simulink model "Hybrid2_article_SVC_stage1"  (R2025a)
settings: Solver=FixedStepAuto  StartTime=0.0  StopTime=0.2  FixedStep=Ts  RelTol=1e-3
undefined symbols (not defined in the file or in its folder): closedLoop, controller, D1, D11, Delta, DiscIntNeverNeededParam, find_system, grid, level, protection, sensor, solarPanel, solarPlant, Ts
libraries: powerlib_extras x38, nesl_utility x29, spsSampleandHoldLib x24, spsThyristorLib x24, spsSeriesRLCBranchLib x23, simulink x22, fl_lib x18, ee_lib x12, spsEdgeDetectorLib x12, spsParallelRLCBranchLib x10, spsThreePhaseVIMeasurementLib x9, simulink_extras x8
(part 7 of 8)

== system Hybrid2_article_SVC_stage1/SVC Controller1/Firing Unit/Firing Unit BC/TCR Pulse Generatorr ==
  Ns/c : Inport
  Alpha : Inport  Port=2  PortDimensions=1
  Sync +/- : Inport  Port=3  PortDimensions=1
  SqWave : Inport  Port=4  PortDimensions=1
  Alpha 90<A<181 : Constant  Value=90
  Alpha 90<A<182 : Constant  Value=360
  Alpha 90<A<183 : Constant  Value=2
  Alpha 90<A<184 : Constant  Value=2
  Alpha 90<A<185 : Constant  Value=87
  Data Type Conversion : DataTypeConversion  OutDataTypeStr=double  SaturateOnIntegerOverflow=off  RndMeth=Floor
  Discrete-Time Integrator : DiscreteIntegrator  ExternalReset=rising  SampleTime=Ts  LimitOutput=on  UpperSaturationLimit=100000  LowerSaturationLimit=0  ICPrevOutput=DiscIntNeverNeededParam  ICPrevScaledInput=DiscIntNeverNeededParam
  Gain2 : Gain  Gain=1/Ts  OutDataTypeStr=double  SaturateOnIntegerOverflow=on  ParamDataTypeStr=Inherit: Same as input
  Logical Operator1 : Logic  Inputs=3
  Logical Operator2 : Logic  Operator=NOT  Inputs=3
  Product : Product  Inputs=*/  InputSameDT=on  SaturateOnIntegerOverflow=on  OutDataTypeStr=Inherit: Same as first input
  Product1 : Product  Inputs=**  InputSameDT=on  SaturateOnIntegerOverflow=on  OutDataTypeStr=Inherit: Same as first input
  Product2 : Product  Inputs=*/  InputSameDT=on  SaturateOnIntegerOverflow=on  OutDataTypeStr=Inherit: Same as first input
  Relational Operator1 : RelationalOperator  Operator=<=
  Relational Operator2 : RelationalOperator
  Relational Operator3 : RelationalOperator  Operator=<=
  Rounding Function1 : Rounding  Operator=round
  Rounding Function3 : Rounding  Operator=round
  Sample and Hold : spsSampleandHoldLib/Sample and Hold  ic=180  Ts=Ts
      settings: AttributesFormatString=IC = %<ic>
  Sum1 : Sum  Inputs=+-  InputSameDT=on  SaturateOnIntegerOverflow=on  OutDataTypeStr=Inherit: Same as first input
  Sum2 : Sum  Inputs=+--  InputSameDT=on  SaturateOnIntegerOverflow=on  OutDataTypeStr=Inherit: Same as first input
  Switch : Switch  Criteria=u2 > Threshold
  TCR +/- : Outport  VectorParamsAs1DForOutWhenUnconnected=off
  wires:
  Alpha 90<A<181/1 -> Sum1/2
  Ns/c/1 -> Product1/1, Product2/1
  Product1/1 -> Rounding Function1/1
  Alpha 90<A<182/1 -> Product/2
  Product/1 -> Product1/2
  Product2/1 -> Rounding Function3/1
  Alpha 90<A<183/1 -> Product2/2
  Sum1/1 -> Product/1, Relational Operator1/1
  Alpha 90<A<185/1 -> Relational Operator1/2
  Alpha/1 -> Sample and Hold/1
  Rounding Function1/1 -> Sum2/3, Switch/1
  Rounding Function3/1 -> Sum2/1, Switch/3
  Alpha 90<A<184/1 -> Sum2/2
  Relational Operator1/1 -> Switch/2
  Relational Operator3/1 -> Logical Operator1/3
  Discrete-Time Integrator/1 -> Relational Operator2/1, Relational Operator3/1
  Relational Operator2/1 -> Logical Operator1/2
  Logical Operator1/1 -> TCR +/-/1
  Switch/1 -> Relational Operator2/2
  Sum2/1 -> Relational Operator3/2
  Logical Operator2/1 -> Discrete-Time Integrator/2
  SqWave/1 -> Data Type Conversion/1, Logical Operator2/1, Logical Operator1/1
  Sync +/-/1 -> Sample and Hold/2
  Sample and Hold/1 -> Sum1/1
  Data Type Conversion/1 -> Gain2/1
  Gain2/1 -> Discrete-Time Integrator/1

== system Hybrid2_article_SVC_stage1/SVC Controller1/Firing Unit/Firing Unit BC/TCR Pulse Generatorr1 ==
  Ns/c : Inport
  Alpha : Inport  Port=2  PortDimensions=1
  Sync +/- : Inport  Port=3  PortDimensions=1
  SqWave : Inport  Port=4  PortDimensions=1
  Alpha 90<A<181 : Constant  Value=90
  Alpha 90<A<182 : Constant  Value=360
  Alpha 90<A<183 : Constant  Value=2
  Alpha 90<A<184 : Constant  Value=2
  Alpha 90<A<185 : Constant  Value=87
  Data Type Conversion : DataTypeConversion  OutDataTypeStr=double  SaturateOnIntegerOverflow=off  RndMeth=Floor
  Discrete-Time Integrator : DiscreteIntegrator  ExternalReset=rising  SampleTime=Ts  OutDataTypeStr=double  LimitOutput=on  UpperSaturationLimit=100000  LowerSaturationLimit=0  ICPrevOutput=DiscIntNeverNeededParam  ICPrevScaledInput=DiscIntNeverNeededParam
  Gain2 : Gain  Gain=1/Ts  OutDataTypeStr=double  ParamDataTypeStr=Inherit: Same as input
  Logical Operator1 : Logic  Inputs=3
  Logical Operator2 : Logic  Operator=NOT  Inputs=3
  Product : Product  Inputs=*/  InputSameDT=on  SaturateOnIntegerOverflow=on  OutDataTypeStr=Inherit: Same as first input
  Product1 : Product  Inputs=**  InputSameDT=on  SaturateOnIntegerOverflow=on  OutDataTypeStr=Inherit: Same as first input
  Product2 : Product  Inputs=*/  InputSameDT=on  SaturateOnIntegerOverflow=on  OutDataTypeStr=Inherit: Same as first input
  Relational Operator1 : RelationalOperator  Operator=<=
  Relational Operator2 : RelationalOperator
  Relational Operator3 : RelationalOperator  Operator=<=
  Rounding Function1 : Rounding  Operator=round
  Rounding Function3 : Rounding  Operator=round
  Sample and Hold : spsSampleandHoldLib/Sample and Hold  ic=180  Ts=Ts
      settings: AttributesFormatString=IC = %<ic>
  Sum1 : Sum  Inputs=+-  InputSameDT=on  SaturateOnIntegerOverflow=on  OutDataTypeStr=Inherit: Same as first input
  Sum2 : Sum  Inputs=+--  OutDataTypeStr=Inherit: Inherit via back propagation  InputSameDT=on  SaturateOnIntegerOverflow=on
  Switch : Switch  Criteria=u2 > Threshold  OutDataTypeStr=Inherit: Inherit via back propagation
  TCR +/- : Outport  VectorParamsAs1DForOutWhenUnconnected=off
  wires:
  Alpha 90<A<181/1 -> Sum1/2
  Ns/c/1 -> Product1/1, Product2/1
  Product1/1 -> Rounding Function1/1
  Alpha 90<A<182/1 -> Product/2
  Product/1 -> Product1/2
  Product2/1 -> Rounding Function3/1
  Alpha 90<A<183/1 -> Product2/2
  Sum1/1 -> Product/1, Relational Operator1/1
  Alpha 90<A<185/1 -> Relational Operator1/2
  Alpha/1 -> Sample and Hold/1
  Rounding Function1/1 -> Sum2/3, Switch/1
  Rounding Function3/1 -> Sum2/1, Switch/3
  Alpha 90<A<184/1 -> Sum2/2
  Relational Operator1/1 -> Switch/2
  Relational Operator3/1 -> Logical Operator1/3
  Discrete-Time Integrator/1 -> Relational Operator2/1, Relational Operator3/1
  Relational Operator2/1 -> Logical Operator1/2
  Logical Operator1/1 -> TCR +/-/1
  Gain2/1 -> Discrete-Time Integrator/1
  Switch/1 -> Relational Operator2/2
  Sum2/1 -> Relational Operator3/2
  Logical Operator2/1 -> Discrete-Time Integrator/2
  SqWave/1 -> Data Type Conversion/1, Logical Operator1/1, Logical Operator2/1
  Sync +/-/1 -> Sample and Hold/2
  Sample and Hold/1 -> Sum1/1
  Data Type Conversion/1 -> Gain2/1

== system Hybrid2_article_SVC_stage1/SVC Controller1/Firing Unit/Firing Unit BC/TCS Pulse Generator ==
  note: Note: Sync+ , Sync - and SqWave signals are inverted for TSC firing (i.e. positive thyristor is fired on negative peak voltage)
  SqWave : Inport  PortDimensions=1
  Sync + : Inport  Port=2  PortDimensions=1
  Sync - : Inport  Port=3  PortDimensions=1
  TSC_On : Inport  Port=4  PortDimensions=1
  Alpha1 : Constant  Value=FiringMode-1  OutDataTypeStr=Inherit: Inherit via back propagation
  Delay : Delay  DelayLength=fix(1/FreqInit/Ts)
  Logical Operator1 : Logic  Operator=NOT
  Logical Operator10 : Logic  Operator=OR
  Logical Operator11 : Logic  Inputs=3
  Logical Operator12 : Logic
  Logical Operator13 : Logic
  Logical Operator14 : Logic  Operator=OR
  Logical Operator15 : Logic  Inputs=3
  Sample and Hold : spsSampleandHoldLib/Sample and Hold  ic=0  Ts=Ts
      settings: AttributesFormatString=IC = %<ic>
  Sample and Hold1 : spsSampleandHoldLib/Sample and Hold  ic=0  Ts=Ts
      settings: AttributesFormatString=IC = %<ic>
  TSC + : Outport  VectorParamsAs1DForOutWhenUnconnected=off
  TSC - : Outport  Port=2  VectorParamsAs1DForOutWhenUnconnected=off
  wires:
  Delay/1 -> Logical Operator14/2, Logical Operator10/2
  Logical Operator15/1 -> TSC -/1
  Logical Operator11/1 -> TSC +/1
  Logical Operator14/1 -> Logical Operator15/2
  Logical Operator10/1 -> Logical Operator11/2
  Logical Operator1/1 -> Logical Operator10/1
  SqWave/1 -> Logical Operator14/1, Logical Operator1/1
  Logical Operator12/1 -> Delay/1
  Alpha1/1 -> Logical Operator12/2
  Logical Operator13/1 -> Logical Operator12/1
  TSC_On/1 -> Sample and Hold1/1, Sample and Hold/1, Logical Operator15/3, Logical Operator11/3
  Sync -/1 -> Sample and Hold/2
  Sync +/1 -> Sample and Hold1/2
  Sample and Hold/1 -> Logical Operator13/1, Logical Operator11/1
  Sample and Hold1/1 -> Logical Operator13/2, Logical Operator15/1

== system Hybrid2_article_SVC_stage1/SVC Controller1/Firing Unit/Firing Unit BC/TCS Pulse Generator1 ==
  note: Note: Sync+ , Sync - and SqWave signals are inverted for TSC firing (i.e. positive thyristor is fired on negative peak voltage)
  SqWave : Inport  PortDimensions=1
  Sync + : Inport  Port=2  PortDimensions=1
  Sync - : Inport  Port=3  PortDimensions=1
  TSC_On : Inport  Port=4  PortDimensions=1
  Alpha1 : Constant  Value=FiringMode-1
  Data Type Conversion : DataTypeConversion  OutDataTypeStr=boolean  SaturateOnIntegerOverflow=off  RndMeth=Floor
  Delay : Delay  DelayLength=fix(1/FreqInit/Ts)
  Logical Operator1 : Logic  Operator=NOT
  Logical Operator10 : Logic  Operator=OR
  Logical Operator11 : Logic  Inputs=3
  Logical Operator12 : Logic
  Logical Operator13 : Logic
  Logical Operator14 : Logic  Operator=OR
  Logical Operator15 : Logic  Inputs=3
  Sample and Hold : spsSampleandHoldLib/Sample and Hold  ic=0  Ts=Ts
      settings: AttributesFormatString=IC = %<ic>
  Sample and Hold1 : spsSampleandHoldLib/Sample and Hold  ic=0  Ts=Ts
      settings: AttributesFormatString=IC = %<ic>
  TSC + : Outport  VectorParamsAs1DForOutWhenUnconnected=off
  TSC - : Outport  Port=2  VectorParamsAs1DForOutWhenUnconnected=off
  wires:
  Delay/1 -> Logical Operator14/2, Logical Operator10/2
  Logical Operator15/1 -> TSC -/1
  Logical Operator11/1 -> TSC +/1
  Logical Operator14/1 -> Logical Operator15/2
  Logical Operator10/1 -> Logical Operator11/2
  Logical Operator1/1 -> Logical Operator10/1
  SqWave/1 -> Logical Operator14/1, Logical Operator1/1
  Logical Operator12/1 -> Delay/1
  Logical Operator13/1 -> Logical Operator12/1
  TSC_On/1 -> Sample and Hold1/1, Sample and Hold/1, Logical Operator15/3, Logical Operator11/3
  Sync -/1 -> Sample and Hold/2
  Sync +/1 -> Sample and Hold1/2
  Sample and Hold/1 -> Logical Operator13/1, Logical Operator11/1
  Sample and Hold1/1 -> Logical Operator13/2, Logical Operator15/1
  Alpha1/1 -> Data Type Conversion/1
  Data Type Conversion/1 -> Logical Operator12/2

== system Hybrid2_article_SVC_stage1/SVC Controller1/Firing Unit/Firing Unit BC/TCS Pulse Generator2 ==
  note: Note: Sync+ , Sync - and SqWave signals are inverted for TSC firing (i.e. positive thyristor is fired on negative peak voltage)
  SqWave : Inport  PortDimensions=1
  Sync + : Inport  Port=2  PortDimensions=1
  Sync - : Inport  Port=3  PortDimensions=1
  TSC_On : Inport  Port=4  PortDimensions=1
  Alpha1 : Constant  Value=FiringMode-1
  Data Type Conversion : DataTypeConversion  OutDataTypeStr=boolean  SaturateOnIntegerOverflow=off  RndMeth=Floor
  Delay : Delay  DelayLength=fix(1/FreqInit/Ts)
  Logical Operator1 : Logic  Operator=NOT
  Logical Operator10 : Logic  Operator=OR
  Logical Operator11 : Logic  Inputs=3
  Logical Operator12 : Logic
  Logical Operator13 : Logic
  Logical Operator14 : Logic  Operator=OR
  Logical Operator15 : Logic  Inputs=3
  Sample and Hold : spsSampleandHoldLib/Sample and Hold  ic=0  Ts=Ts
      settings: AttributesFormatString=IC = %<ic>
  Sample and Hold1 : spsSampleandHoldLib/Sample and Hold  ic=0  Ts=Ts
      settings: AttributesFormatString=IC = %<ic>
  TSC + : Outport  VectorParamsAs1DForOutWhenUnconnected=off
  TSC - : Outport  Port=2  VectorParamsAs1DForOutWhenUnconnected=off
  wires:
  Delay/1 -> Logical Operator14/2, Logical Operator10/2
  Logical Operator15/1 -> TSC -/1
  Logical Operator11/1 -> TSC +/1
  Logical Operator14/1 -> Logical Operator15/2
  Logical Operator10/1 -> Logical Operator11/2
  Logical Operator1/1 -> Logical Operator10/1
  SqWave/1 -> Logical Operator14/1, Logical Operator1/1
  Logical Operator12/1 -> Delay/1
  Alpha1/1 -> Data Type Conversion/1
  Logical Operator13/1 -> Logical Operator12/1
  TSC_On/1 -> Sample and Hold1/1, Sample and Hold/1, Logical Operator15/3, Logical Operator11/3
  Sync -/1 -> Sample and Hold/2
  Sync +/1 -> Sample and Hold1/2
  Sample and Hold/1 -> Logical Operator13/1, Logical Operator11/1
  Sample and Hold1/1 -> Logical Operator13/2, Logical Operator15/1
  Data Type Conversion/1 -> Logical Operator12/2

== system Hybrid2_article_SVC_stage1/SVC Controller1/Firing Unit/Firing Unit CA/BL2 ==
  Freq : Inport  PortDimensions=1
  Constant1 : Constant  Value=0
  Constant2 : Constant  Value=1e-5
  Constant3 : Constant
  Gain : Gain  Gain=Ts  SaturateOnIntegerOverflow=on  OutDataTypeStr=Inherit: Same as input  ParamDataTypeStr=Inherit: Same as input
  Product : Product  Inputs=/*  InputSameDT=on  SaturateOnIntegerOverflow=on  OutDataTypeStr=Inherit: Same as first input
  Relational Operator1 : RelationalOperator  Operator=~=
  Switch : Switch  Threshold=0.5
  Ns/c : Outport  VectorParamsAs1DForOutWhenUnconnected=off
  wires:
  Product/1 -> Ns/c/1
  Freq/1 -> Gain/1
  Constant1/1 -> Relational Operator1/2
  Gain/1 -> Relational Operator1/1, Switch/1
  Constant2/1 -> Switch/3
  Relational Operator1/1 -> Switch/2
  Switch/1 -> Product/1
  Constant3/1 -> Product/2

== system Hybrid2_article_SVC_stage1/SVC Controller1/Firing Unit/Firing Unit CA/BL3 ==
  Freq : Inport  PortDimensions=1
  sin(wt) : Inport  Port=2  PortDimensions=1
  Bistable : spsBistableLib/Bistable  Qpriority=Set  ic=0  Ts=Ts
  Data Type Conversion : DataTypeConversion  SaturateOnIntegerOverflow=off  RndMeth=Floor
  Edge Detector : spsEdgeDetectorLib/Edge Detector  model=Rising  ic=0  Ts=Ts
  Edge Detector1 : spsEdgeDetectorLib/Edge Detector  model=Falling  ic=0  Ts=Ts
  Edge Detector2 : spsEdgeDetectorLib/Edge Detector  model=Rising  ic=0  Ts=Ts
  Edge Detector3 : spsEdgeDetectorLib/Edge Detector  model=Rising  ic=0  Ts=Ts
  Product2 : Product  InputSameDT=on  SaturateOnIntegerOverflow=on  OutDataTypeStr=Inherit: Same as first input
  Relational Operator : RelationalOperator  Operator=>
  Relational Operator2 : RelationalOperator  Operator=<
  Sum5 : Sum  Inputs=+-  InputSameDT=on  SaturateOnIntegerOverflow=on  OutDataTypeStr=Inherit: Same as first input
  Sum6 : Sum  InputSameDT=on  SaturateOnIntegerOverflow=on  OutDataTypeStr=Inherit: Same as first input
  Terminator : Terminator
  Trigonometric Function7 : Trigonometry
  alpha2 : Constant  Value=0
  alpha9 : Constant  Value=pi*Ts
  SqWave : Outport  VectorParamsAs1DForOutWhenUnconnected=off
  Sync + : Outport  Port=2  VectorParamsAs1DForOutWhenUnconnected=off
  Sync - : Outport  Port=3  VectorParamsAs1DForOutWhenUnconnected=off
  wires:
  Data Type Conversion/1 -> Edge Detector/1, Edge Detector1/1, SqWave/1
  Bistable/2 -> Terminator/1
  Edge Detector3/1 -> Bistable/2
  Edge Detector2/1 -> Bistable/1
  Edge Detector1/1 -> Sync -/1
  Edge Detector/1 -> Sync +/1
  Bistable/1 -> Data Type Conversion/1
  alpha9/1 -> Product2/1
  Product2/1 -> Trigonometric Function7/1
  Relational Operator2/1 -> Edge Detector3/1
  Relational Operator/1 -> Edge Detector2/1
  Sum6/1 -> Relational Operator2/2
  Sum5/1 -> Relational Operator/2
  alpha2/1 -> Sum6/1, Sum5/1
  Trigonometric Function7/1 -> Sum6/2, Sum5/2
  Freq/1 -> Product2/2
  sin(wt)/1 -> Relational Operator/1, Relational Operator2/1

== system Hybrid2_article_SVC_stage1/SVC Controller1/Firing Unit/Firing Unit CA/PLL sync on positive peak  ==
  note: Note: -sin( a ) * sin( b ) = 1/2 * cos( a+b ) - 1/2 * cos(a-b)
  note: Discrete 1-phase PLL
  note: Note: PLL synchronized on positive peak of input
  note: Pierre Giroux, Gilbert Sybille
      | Power System Laboratory, IREQ
      | Hydro-Quebec
  V(pu) : Inport
  Constant4 : Constant  Value=2*pi
  Discrete PI Controller : Subsystem  DialogController=POWERSYS.PowerSysDialog  mask(Discrete PI Controller){Kp=Kp, Ki=Ki, Par_Limits=[1.25  0.75]*2*pi*Finit, Init=2*pi*Finit, Ts=Ts}
      mask prompts: Kp "Proportional gain (Kp):"; Ki "Integral gain (Ki):"; Par_Limits "Output limits: [ Upper   Lower ]"; Init "Output initial value:"; Ts "Sample time:"
      mask help: This block implements a discrete PI controller.
      mask init:
      | UpperLimit=Par_Limits(1);
      | LowerLimit=Par_Limits(2);
      | power_initmask();
      mask Help: This block is part of a subset of blocks in the Extras library that does not have documentation associated with it, other than the block mask description.
      mask Display: disp('PI');
  Discrete-Time Integrator : DiscreteIntegrator  InitialCondition=(Phase_Init-90)*pi/180  SampleTime=Ts  ICPrevOutput=DiscIntNeverNeededParam  ICPrevScaledInput=DiscIntNeverNeededParam
  Gain10 : Gain  Gain=1/2/pi  SaturateOnIntegerOverflow=on  OutDataTypeStr=Inherit: Same as input  ParamDataTypeStr=Inherit: Same as input
  Gain12 : Gain  Gain=-1  SaturateOnIntegerOverflow=on  OutDataTypeStr=Inherit: Same as input  ParamDataTypeStr=Inherit: Same as input
  Math Function : Math  Operator=mod  SignedPower=on
  Mean (Variable Frequency)1 : spsMeanVariableFrequencyLib/Mean (Variable Frequency)  Finit=Finit  Fmin=45  Vinit=0  Ts=Ts
  Product1 : Product  InputSameDT=on  SaturateOnIntegerOverflow=on  OutDataTypeStr=Inherit: Same as first input
  Rate Limiter : RateLimiter  RisingSlewLimit=10  FallingSlewLimit=-10  SampleTimeMode=inherited  InitialCondition=Finit
  Second-Order Filter : spsSecondOrderFilterLib/Second-Order Filter  FilterType=Lowpass  Fo=25  Zeta=0.707  Ts=Ts  Initialize=on  Vac_Init="[0 0  Finit]"  Vdc_Init=Finit  PlotResponse=off  FreqRange=[1 500 1]
  Trigonometric Function6 : Trigonometry
  Unit Delay1 : UnitDelay  InitialCondition=Finit  SampleTime=Ts  HasFrameUpgradeWarning=on
      settings: AttributesFormatString=IC = %<InitialCondition>
  Freq : Outport  VectorParamsAs1DForOutWhenUnconnected=off
  wt : Outport  Port=2  VectorParamsAs1DForOutWhenUnconnected=off
  wires:
  Gain12/1 -> Product1/1
  V(pu)/1 -> Gain12/1
  Constant4/1 -> Math Function/2
  Discrete-Time Integrator/1 -> Math Function/1
  Product1/1 -> Mean (Variable Frequency)1/2
  Discrete PI Controller/1(Out) -> Discrete-Time Integrator/1, Gain10/1  "W"
  Gain10/1 -> Rate Limiter/1
  Rate Limiter/1 -> Second-Order Filter/1
  Second-Order Filter/1 -> Unit Delay1/1
  Trigonometric Function6/1 -> Product1/2
  Math Function/1 -> Trigonometric Function6/1, wt/1
  Unit Delay1/1 -> Mean (Variable Frequency)1/1, Freq/1
  Mean (Variable Frequency)1/1 -> Discrete PI Controller/1(Error)

== system Hybrid2_article_SVC_stage1/SVC Controller1/Firing Unit/Firing Unit CA/TCR Pulse Generatorr ==
  Ns/c : Inport
  Alpha : Inport  Port=2  PortDimensions=1
  Sync +/- : Inport  Port=3  PortDimensions=1
  SqWave : Inport  Port=4  PortDimensions=1
  Alpha 90<A<181 : Constant  Value=90
  Alpha 90<A<182 : Constant  Value=360
  Alpha 90<A<183 : Constant  Value=2
  Alpha 90<A<184 : Constant  Value=2
  Alpha 90<A<185 : Constant  Value=87
  Data Type Conversion : DataTypeConversion  OutDataTypeStr=double  SaturateOnIntegerOverflow=off  RndMeth=Floor
  Discrete-Time Integrator : DiscreteIntegrator  ExternalReset=rising  SampleTime=Ts  LimitOutput=on  UpperSaturationLimit=100000  LowerSaturationLimit=0  ICPrevOutput=DiscIntNeverNeededParam  ICPrevScaledInput=DiscIntNeverNeededParam
  Gain2 : Gain  Gain=1/Ts  OutDataTypeStr=double  ParamDataTypeStr=Inherit: Same as input
  Logical Operator1 : Logic  Inputs=3
  Logical Operator2 : Logic  Operator=NOT  Inputs=3
  Product : Product  Inputs=*/  InputSameDT=on  SaturateOnIntegerOverflow=on  OutDataTypeStr=Inherit: Same as first input
  Product1 : Product  Inputs=**  InputSameDT=on  SaturateOnIntegerOverflow=on  OutDataTypeStr=Inherit: Same as first input
  Product2 : Product  Inputs=*/  InputSameDT=on  SaturateOnIntegerOverflow=on  OutDataTypeStr=Inherit: Same as first input
  Relational Operator1 : RelationalOperator  Operator=<=
  Relational Operator2 : RelationalOperator
  Relational Operator3 : RelationalOperator  Operator=<=
  Rounding Function1 : Rounding  Operator=round
  Rounding Function3 : Rounding  Operator=round
  Sample and Hold : spsSampleandHoldLib/Sample and Hold  ic=180  Ts=Ts
      settings: AttributesFormatString=IC = %<ic>
  Sum1 : Sum  Inputs=+-  InputSameDT=on  SaturateOnIntegerOverflow=on  OutDataTypeStr=Inherit: Same as first input
  Sum2 : Sum  Inputs=+--  InputSameDT=on  SaturateOnIntegerOverflow=on  OutDataTypeStr=Inherit: Same as first input
  Switch : Switch  Criteria=u2 > Threshold
  TCR +/- : Outport  VectorParamsAs1DForOutWhenUnconnected=off
  wires:
  Alpha 90<A<181/1 -> Sum1/2
  Ns/c/1 -> Product1/1, Product2/1
  Product1/1 -> Rounding Function1/1
  Alpha 90<A<182/1 -> Product/2
  Product/1 -> Product1/2
  Product2/1 -> Rounding Function3/1
  Alpha 90<A<183/1 -> Product2/2
  Sum1/1 -> Product/1, Relational Operator1/1
  Alpha 90<A<185/1 -> Relational Operator1/2
  Alpha/1 -> Sample and Hold/1
  Rounding Function1/1 -> Sum2/3, Switch/1
  Rounding Function3/1 -> Sum2/1, Switch/3
  Alpha 90<A<184/1 -> Sum2/2
  Relational Operator1/1 -> Switch/2
  Relational Operator3/1 -> Logical Operator1/3
  Discrete-Time Integrator/1 -> Relational Operator2/1, Relational Operator3/1
  Relational Operator2/1 -> Logical Operator1/2
  Logical Operator1/1 -> TCR +/-/1
  Switch/1 -> Relational Operator2/2
  Sum2/1 -> Relational Operator3/2
  Logical Operator2/1 -> Discrete-Time Integrator/2
  SqWave/1 -> Data Type Conversion/1, Logical Operator1/1, Logical Operator2/1
  Sync +/-/1 -> Sample and Hold/2
  Sample and Hold/1 -> Sum1/1
  Data Type Conversion/1 -> Gain2/1
  Gain2/1 -> Discrete-Time Integrator/1

== system Hybrid2_article_SVC_stage1/SVC Controller1/Firing Unit/Firing Unit CA/TCR Pulse Generatorr1 ==
  Ns/c : Inport
  Alpha : Inport  Port=2  PortDimensions=1
  Sync +/- : Inport  Port=3  PortDimensions=1
  SqWave : Inport  Port=4  PortDimensions=1
  Alpha 90<A<181 : Constant  Value=90
  Alpha 90<A<182 : Constant  Value=360
  Alpha 90<A<183 : Constant  Value=2
  Alpha 90<A<184 : Constant  Value=2
  Alpha 90<A<185 : Constant  Value=87
  Data Type Conversion : DataTypeConversion  OutDataTypeStr=double  SaturateOnIntegerOverflow=off  RndMeth=Floor
  Discrete-Time Integrator : DiscreteIntegrator  ExternalReset=rising  SampleTime=Ts  OutDataTypeStr=double  LimitOutput=on  UpperSaturationLimit=100000  LowerSaturationLimit=0  ICPrevOutput=DiscIntNeverNeededParam  ICPrevScaledInput=DiscIntNeverNeededParam
  Gain2 : Gain  Gain=1/Ts  OutDataTypeStr=double  ParamDataTypeStr=Inherit: Same as input
  Logical Operator1 : Logic  Inputs=3
  Logical Operator2 : Logic  Operator=NOT  Inputs=3
  Product : Product  Inputs=*/  InputSameDT=on  SaturateOnIntegerOverflow=on  OutDataTypeStr=Inherit: Same as first input
  Product1 : Product  Inputs=**  InputSameDT=on  SaturateOnIntegerOverflow=on  OutDataTypeStr=Inherit: Same as first input
  Product2 : Product  Inputs=*/  InputSameDT=on  SaturateOnIntegerOverflow=on  OutDataTypeStr=Inherit: Same as first input
  Relational Operator1 : RelationalOperator  Operator=<=
  Relational Operator2 : RelationalOperator
  Relational Operator3 : RelationalOperator  Operator=<=
  Rounding Function1 : Rounding  Operator=round
  Rounding Function3 : Rounding  Operator=round
  Sample and Hold : spsSampleandHoldLib/Sample and Hold  ic=180  Ts=Ts
      settings: AttributesFormatString=IC = %<ic>
  Sum1 : Sum  Inputs=+-  InputSameDT=on  SaturateOnIntegerOverflow=on  OutDataTypeStr=Inherit: Same as first input
  Sum2 : Sum  Inputs=+--  OutDataTypeStr=Inherit: Inherit via back propagation  InputSameDT=on  SaturateOnIntegerOverflow=on
  Switch : Switch  Criteria=u2 > Threshold  OutDataTypeStr=Inherit: Inherit via back propagation
  TCR +/- : Outport  VectorParamsAs1DForOutWhenUnconnected=off
  wires:
  Alpha 90<A<181/1 -> Sum1/2
  Ns/c/1 -> Product1/1, Product2/1
  Product1/1 -> Rounding Function1/1
  Alpha 90<A<182/1 -> Product/2
  Product/1 -> Product1/2
  Product2/1 -> Rounding Function3/1
  Alpha 90<A<183/1 -> Product2/2
  Sum1/1 -> Product/1, Relational Operator1/1
  Alpha 90<A<185/1 -> Relational Operator1/2
  Alpha/1 -> Sample and Hold/1
  Rounding Function1/1 -> Sum2/3, Switch/1
  Rounding Function3/1 -> Sum2/1, Switch/3
  Alpha 90<A<184/1 -> Sum2/2
  Relational Operator1/1 -> Switch/2
  Relational Operator3/1 -> Logical Operator1/3
  Discrete-Time Integrator/1 -> Relational Operator2/1, Relational Operator3/1
  Relational Operator2/1 -> Logical Operator1/2
  Logical Operator1/1 -> TCR +/-/1
  Gain2/1 -> Discrete-Time Integrator/1
  Switch/1 -> Relational Operator2/2
  Sum2/1 -> Relational Operator3/2
  Logical Operator2/1 -> Discrete-Time Integrator/2
  SqWave/1 -> Data Type Conversion/1, Logical Operator1/1, Logical Operator2/1
  Sync +/-/1 -> Sample and Hold/2
  Sample and Hold/1 -> Sum1/1
  Data Type Conversion/1 -> Gain2/1

== system Hybrid2_article_SVC_stage1/SVC Controller1/Firing Unit/Firing Unit CA/TCS Pulse Generator ==
  note: Note: Sync+ , Sync - and SqWave signals are inverted for TSC firing (i.e. positive thyristor is fired on negative peak voltage)
  SqWave : Inport  PortDimensions=1
  Sync + : Inport  Port=2  PortDimensions=1
  Sync - : Inport  Port=3  PortDimensions=1
  TSC_On : Inport  Port=4  PortDimensions=1
  Alpha1 : Constant  Value=FiringMode-1  OutDataTypeStr=boolean
  Delay : Delay  DelayLength=fix(1/FreqInit/Ts)
  Logical Operator1 : Logic  Operator=NOT
  Logical Operator10 : Logic  Operator=OR
  Logical Operator11 : Logic  Inputs=3
  Logical Operator12 : Logic
  Logical Operator13 : Logic
  Logical Operator14 : Logic  Operator=OR
  Logical Operator15 : Logic  Inputs=3
  Sample and Hold : spsSampleandHoldLib/Sample and Hold  ic=0  Ts=Ts
      settings: AttributesFormatString=IC = %<ic>
  Sample and Hold1 : spsSampleandHoldLib/Sample and Hold  ic=0  Ts=Ts
      settings: AttributesFormatString=IC = %<ic>
  TSC + : Outport  VectorParamsAs1DForOutWhenUnconnected=off
  TSC - : Outport  Port=2  VectorParamsAs1DForOutWhenUnconnected=off
  wires:
  Delay/1 -> Logical Operator14/2, Logical Operator10/2
  Logical Operator15/1 -> TSC -/1
  Logical Operator11/1 -> TSC +/1
  Logical Operator14/1 -> Logical Operator15/2
  Logical Operator10/1 -> Logical Operator11/2
  Logical Operator1/1 -> Logical Operator10/1
  SqWave/1 -> Logical Operator14/1, Logical Operator1/1
  Logical Operator12/1 -> Delay/1
  Alpha1/1 -> Logical Operator12/2
  Logical Operator13/1 -> Logical Operator12/1
  TSC_On/1 -> Sample and Hold1/1, Sample and Hold/1, Logical Operator15/3, Logical Operator11/3
  Sync -/1 -> Sample and Hold/2
  Sync +/1 -> Sample and Hold1/2
  Sample and Hold/1 -> Logical Operator13/1, Logical Operator11/1
  Sample and Hold1/1 -> Logical Operator13/2, Logical Operator15/1

== system Hybrid2_article_SVC_stage1/SVC Controller1/Firing Unit/Firing Unit CA/TCS Pulse Generator1 ==
  note: Note: Sync+ , Sync - and SqWave signals are inverted for TSC firing (i.e. positive thyristor is fired on negative peak voltage)
  SqWave : Inport  PortDimensions=1
  Sync + : Inport  Port=2  PortDimensions=1
  Sync - : Inport  Port=3  PortDimensions=1
  TSC_On : Inport  Port=4  PortDimensions=1
  Alpha1 : Constant  Value=FiringMode-1
  Data Type Conversion : DataTypeConversion  OutDataTypeStr=boolean  SaturateOnIntegerOverflow=off  RndMeth=Floor  LockScale=on
  Delay : Delay  DelayLength=fix(1/FreqInit/Ts)
  Logical Operator1 : Logic  Operator=NOT
  Logical Operator10 : Logic  Operator=OR
  Logical Operator11 : Logic  Inputs=3
  Logical Operator12 : Logic
  Logical Operator13 : Logic
  Logical Operator14 : Logic  Operator=OR
  Logical Operator15 : Logic  Inputs=3
  Sample and Hold : spsSampleandHoldLib/Sample and Hold  ic=0  Ts=Ts
      settings: AttributesFormatString=IC = %<ic>
  Sample and Hold1 : spsSampleandHoldLib/Sample and Hold  ic=0  Ts=Ts
      settings: AttributesFormatString=IC = %<ic>
  TSC + : Outport  VectorParamsAs1DForOutWhenUnconnected=off
  TSC - : Outport  Port=2  VectorParamsAs1DForOutWhenUnconnected=off
  wires:
  Delay/1 -> Logical Operator14/2, Logical Operator10/2
  Logical Operator15/1 -> TSC -/1
  Logical Operator11/1 -> TSC +/1
  Logical Operator14/1 -> Logical Operator15/2
  Logical Operator10/1 -> Logical Operator11/2
  Logical Operator1/1 -> Logical Operator10/1
  SqWave/1 -> Logical Operator14/1, Logical Operator1/1
  Logical Operator12/1 -> Delay/1
  Logical Operator13/1 -> Logical Operator12/1
  TSC_On/1 -> Sample and Hold1/1, Sample and Hold/1, Logical Operator15/3, Logical Operator11/3
  Sync -/1 -> Sample and Hold/2
  Sync +/1 -> Sample and Hold1/2
  Sample and Hold/1 -> Logical Operator13/1, Logical Operator11/1
  Sample and Hold1/1 -> Logical Operator13/2, Logical Operator15/1
  Alpha1/1 -> Data Type Conversion/1
  Data Type Conversion/1 -> Logical Operator12/2

== system Hybrid2_article_SVC_stage1/SVC Controller1/Firing Unit/Firing Unit CA/TCS Pulse Generator2 ==
  note: Note: Sync+ , Sync - and SqWave signals are inverted for TSC firing (i.e. positive thyristor is fired on negative peak voltage)
  SqWave : Inport  PortDimensions=1
  Sync + : Inport  Port=2  PortDimensions=1
  Sync - : Inport  Port=3  PortDimensions=1
  TSC_On : Inport  Port=4  PortDimensions=1
  Alpha1 : Constant  Value=FiringMode-1
  Delay : Delay  DelayLength=fix(1/FreqInit/Ts)
  Logical Operator1 : Logic  Operator=NOT
  Logical Operator10 : Logic  Operator=OR
  Logical Operator11 : Logic  Inputs=3
  Logical Operator12 : Logic  AllPortsSameDT=off
  Logical Operator13 : Logic
  Logical Operator14 : Logic  Operator=OR
  Logical Operator15 : Logic  Inputs=3
  Sample and Hold : spsSampleandHoldLib/Sample and Hold  ic=0  Ts=Ts
      settings: AttributesFormatString=IC = %<ic>
  Sample and Hold1 : spsSampleandHoldLib/Sample and Hold  ic=0  Ts=Ts
      settings: AttributesFormatString=IC = %<ic>
  TSC + : Outport  VectorParamsAs1DForOutWhenUnconnected=off
  TSC - : Outport  Port=2  VectorParamsAs1DForOutWhenUnconnected=off
  wires:
  Delay/1 -> Logical Operator14/2, Logical Operator10/2
  Logical Operator15/1 -> TSC -/1
  Logical Operator11/1 -> TSC +/1
  Logical Operator14/1 -> Logical Operator15/2
  Logical Operator10/1 -> Logical Operator11/2
  Logical Operator1/1 -> Logical Operator10/1
  SqWave/1 -> Logical Operator14/1, Logical Operator1/1
  Logical Operator12/1 -> Delay/1
  Alpha1/1 -> Logical Operator12/2
  Logical Operator13/1 -> Logical Operator12/1
  TSC_On/1 -> Sample and Hold1/1, Sample and Hold/1, Logical Operator15/3, Logical Operator11/3
  Sync -/1 -> Sample and Hold/2
  Sync +/1 -> Sample and Hold1/2
  Sample and Hold/1 -> Logical Operator13/1, Logical Operator11/1
  Sample and Hold1/1 -> Logical Operator13/2, Logical Operator15/1

== system Hybrid2_article_SVC_stage1/DFIG Wind Turbine/Control/Measurement and Transformation/Discrete 3-phase PLL-Driven Positive-Sequence Active & Reactive Power/Discrete 3-phase PLL-Driven Positive-Sequence Fundamental Value ==
  note: Discrete 3-phase PLL-Driven Positive-Sequence Fundamental Value
  note: Pierre Giroux, Gilbert Sybille
      | Power System Simulation Laboratory
      | IREQ, Hydro-Quebc
  Freq : Inport
  Sin_Cos : Inport  Port=2  PortDimensions=2
  abc : Inport  Port=3  PortDimensions=3
  Cartesian to Polar : simulink_extras/Transformations/Cartesian to Polar
  Demux : Demux  Outputs=3
      settings: DisplayOption=none
  Discrete Variable Frequency Mean value1 : Subsystem  mask(Discrete Variable-Frequency Mean Value){Finit=Finit, Fmin=Fmin, Vinit=Imag_Init, Ts=Ts}
      mask prompts: Finit "Initial frequency (Hz):"; Fmin "Minimum frequency (Hz):"; Vinit "Initial input (DC component):"; Ts "Sample time:"
      mask help:
      | This discrete block computes the mean value of the input signal (port In) over a running window of one cycle of a specified frequency (port Freq).
      |
      | For the first cycle of simulation (specified by the parameter "Initial frequency"), the output is held to the value of the  "Initial input" parameter.
      |
      | The value of the parameter "Minimum frequency" is used to determine the buffer size of the "Variable Transport Delay" block found inside this subsystem.
      mask init:
      | MaxDelay=1/Fmin+Ts;
      | power_initmask();
      settings: OpenFcn=power_openblockproxy();
  Discrete Variable Frequency Mean value2 : Subsystem  mask(Discrete Variable-Frequency Mean Value){Finit=Finit, Fmin=Fmin, Vinit=Real_Init, Ts=Ts}
      mask prompts: Finit "Initial frequency (Hz):"; Fmin "Minimum frequency (Hz):"; Vinit "Initial input (DC component):"; Ts "Sample time:"
      mask help:
      | This discrete block computes the mean value of the input signal (port In) over a running window of one cycle of a specified frequency (port Freq).
      |
      | For the first cycle of simulation (specified by the parameter "Initial frequency"), the output is held to the value of the  "Initial input" parameter.
      |
      | The value of the parameter "Minimum frequency" is used to determine the buffer size of the "Variable Transport Delay" block found inside this subsystem.
      mask init:
      | MaxDelay=1/Fmin+Ts;
      | power_initmask();
      settings: OpenFcn=power_openblockproxy();
  Rad->Deg. : Gain  Gain=180/pi  SaturateOnIntegerOverflow=on  OutDataTypeStr=Inherit: Same as input  ParamDataTypeStr=Inherit: Same as input
  Terminator : Terminator
  abc_to_dq0 Transformation : powerlib_extras/Measurements/abc_to_dq0 Transformation
  Mag : Outport  VectorParamsAs1DForOutWhenUnconnected=off
  Phase : Outport  Port=2  VectorParamsAs1DForOutWhenUnconnected=off
  wires:
  Cartesian to Polar/2 -> Rad->Deg./1
  Cartesian to Polar/1 -> Mag/1
  Demux/3 -> Terminator/1
  abc_to_dq0 Transformation/1 -> Demux/1
  abc/1 -> abc_to_dq0 Transformation/1
  Demux/1 -> Discrete Variable Frequency Mean value2/2(In)
  Demux/2 -> Discrete Variable Frequency Mean value1/2(In)
  Discrete Variable Frequency Mean value1/1(Mean) -> Cartesian to Polar/2  "Real"
  Rad->Deg./1 -> Phase/1
  Discrete Variable Frequency Mean value2/1(Mean) -> Cartesian to Polar/1  "Real"
  Freq/1 -> Discrete Variable Frequency Mean value1/1(Freq), Discrete Variable Frequency Mean value2/1(Freq)
  Sin_Cos/1 -> abc_to_dq0 Transformation/2

== system Hybrid2_article_SVC_stage1/DFIG Wind Turbine/Control/Measurement and Transformation/Discrete 3-phase PLL-Driven Positive-Sequence Active & Reactive Power/Discrete 3-phase PLL-Driven Positive-Sequence Fundamental Value2 ==
  note: Pierre Giroux, Gilbert Sybille
      | Power System Simulation Laboratory
      | IREQ, Hydro-Quebc
  note: Discrete 3-phase PLL-Driven Positive-Sequence Fundamental Value
  Freq : Inport
  Sin_Cos : Inport  Port=2  PortDimensions=2
  abc : Inport  Port=3  PortDimensions=3
  Cartesian to Polar : simulink_extras/Transformations/Cartesian to Polar
  Demux : Demux  Outputs=3
      settings: DisplayOption=none
  Discrete Variable Frequency Mean value1 : Subsystem  mask(Discrete Variable-Frequency Mean Value){Finit=Finit, Fmin=Fmin, Vinit=Imag_Init, Ts=Ts}
      mask prompts: Finit "Initial frequency (Hz):"; Fmin "Minimum frequency (Hz):"; Vinit "Initial input (DC component):"; Ts "Sample time:"
      mask help:
      | This discrete block computes the mean value of the input signal (port In) over a running window of one cycle of a specified frequency (port Freq).
      |
      | For the first cycle of simulation (specified by the parameter "Initial frequency"), the output is held to the value of the  "Initial input" parameter.
      |
      | The value of the parameter "Minimum frequency" is used to determine the buffer size of the "Variable Transport Delay" block found inside this subsystem.
      mask init:
      | MaxDelay=1/Fmin+Ts;
      | power_initmask();
      settings: OpenFcn=power_openblockproxy();
  Discrete Variable Frequency Mean value2 : Subsystem  mask(Discrete Variable-Frequency Mean Value){Finit=Finit, Fmin=Fmin, Vinit=Real_Init, Ts=Ts}
      mask prompts: Finit "Initial frequency (Hz):"; Fmin "Minimum frequency (Hz):"; Vinit "Initial input (DC component):"; Ts "Sample time:"
      mask help:
      | This discrete block computes the mean value of the input signal (port In) over a running window of one cycle of a specified frequency (port Freq).
      |
      | For the first cycle of simulation (specified by the parameter "Initial frequency"), the output is held to the value of the  "Initial input" parameter.
      |
      | The value of the parameter "Minimum frequency" is used to determine the buffer size of the "Variable Transport Delay" block found inside this subsystem.
      mask init:
      | MaxDelay=1/Fmin+Ts;
      | power_initmask();
      settings: OpenFcn=power_openblockproxy();
  Rad->Deg. : Gain  Gain=180/pi  SaturateOnIntegerOverflow=on  OutDataTypeStr=Inherit: Same as input  ParamDataTypeStr=Inherit: Same as input
  Terminator : Terminator
  abc_to_dq0 Transformation : powerlib_extras/Measurements/abc_to_dq0 Transformation
  Mag : Outport  VectorParamsAs1DForOutWhenUnconnected=off
  Phase : Outport  Port=2  VectorParamsAs1DForOutWhenUnconnected=off
  wires:
  Sin_Cos/1 -> abc_to_dq0 Transformation/2
  Freq/1 -> Discrete Variable Frequency Mean value2/1(Freq), Discrete Variable Frequency Mean value1/1(Freq)
  Discrete Variable Frequency Mean value2/1(Mean) -> Cartesian to Polar/1  "Real"
  Rad->Deg./1 -> Phase/1
  Discrete Variable Frequency Mean value1/1(Mean) -> Cartesian to Polar/2  "Real"
  Demux/2 -> Discrete Variable Frequency Mean value1/2(In)
  Demux/1 -> Discrete Variable Frequency Mean value2/2(In)
  abc/1 -> abc_to_dq0 Transformation/1
  abc_to_dq0 Transformation/1 -> Demux/1
  Demux/3 -> Terminator/1
  Cartesian to Polar/1 -> Mag/1
  Cartesian to Polar/2 -> Rad->Deg./1

== system Hybrid2_article_SVC_stage1/DFIG Wind Turbine/Control/Rotor-side Controls/INT/S6 ==
  note: Limiter
      | with external
      | limits
  MAX : Inport
  In : Inport  Port=2
  MIN : Inport  Port=3
  MinMax : MinMax  Function=max  Inputs=2  InputSameDT=on  SaturateOnIntegerOverflow=on
  MinMax1 : MinMax  Inputs=2  InputSameDT=on  SaturateOnIntegerOverflow=on
  "  " : Outport  InitialOutput=0  VectorParamsAs1DForOutWhenUnconnected=off
  wires:
  In/1 -> MinMax1/2
  MinMax/1 -> "  "/1
  MIN/1 -> MinMax/1
  MAX/1 -> MinMax1/1
  MinMax1/1 -> MinMax/2

== system Hybrid2_article_SVC_stage1/SVC Controller1/Firing Unit/Firing Unit AB/PLL sync on positive peak /Discrete PI Controller ==
  note: Discrete PID Controller
  note: Pierre Giroux, Gilbert Sybille
      | Power System Simulation Laboratory
      | IREQ, Hydro-Quebc
  Error : Inport  SampleTime=Ts
  Discrete-Time Integrator : DiscreteIntegrator  InitialCondition=Init  SampleTime=Ts  LimitOutput=on  UpperSaturationLimit=UpperLimit  LowerSaturationLimit=LowerLimit  ICPrevOutput=DiscIntNeverNeededParam  ICPrevScaledInput=DiscIntNeverNeededParam
  Kp4 : Gain  Gain=Kp  SaturateOnIntegerOverflow=on  SampleTime=Ts  OutDataTypeStr=Inherit: Same as input  ParamDataTypeStr=Inherit: Same as input
  Kp5 : Gain  Gain=Ki  SaturateOnIntegerOverflow=on  SampleTime=Ts  OutDataTypeStr=Inherit: Same as input  ParamDataTypeStr=Inherit: Same as input
  Saturation2 : Saturate  UpperLimit=UpperLimit  LowerLimit=LowerLimit  SampleTime=Ts
  Sum6 : Sum  InputSameDT=on  SaturateOnIntegerOverflow=on  SampleTime=Ts  OutDataTypeStr=Inherit: Same as first input
  Zero-Order Hold : ZeroOrderHold  SampleTime=Ts
  Out : Outport  SampleTime=Ts  InitialOutput=0  VectorParamsAs1DForOutWhenUnconnected=off
  wires:
  Zero-Order Hold/1 -> Sum6/1
  Saturation2/1 -> Out/1
  Discrete-Time Integrator/1 -> Sum6/2
  Kp4/1 -> Zero-Order Hold/1
  Kp5/1 -> Discrete-Time Integrator/1
  Sum6/1 -> Saturation2/1
  Error/1 -> Kp5/1, Kp4/1

== system Hybrid2_article_SVC_stage1/SVC Controller1/Firing Unit/Firing Unit BC/PLL sync on positive peak /Discrete PI Controller ==
  note: Discrete PID Controller
  note: Pierre Giroux, Gilbert Sybille
      | Power System Simulation Laboratory
      | IREQ, Hydro-Quebc
  Error : Inport  SampleTime=Ts
  Discrete-Time Integrator : DiscreteIntegrator  InitialCondition=Init  SampleTime=Ts  LimitOutput=on  UpperSaturationLimit=UpperLimit  LowerSaturationLimit=LowerLimit  ICPrevOutput=DiscIntNeverNeededParam  ICPrevScaledInput=DiscIntNeverNeededParam
  Kp4 : Gain  Gain=Kp  SaturateOnIntegerOverflow=on  SampleTime=Ts  OutDataTypeStr=Inherit: Same as input  ParamDataTypeStr=Inherit: Same as input
  Kp5 : Gain  Gain=Ki  SaturateOnIntegerOverflow=on  SampleTime=Ts  OutDataTypeStr=Inherit: Same as input  ParamDataTypeStr=Inherit: Same as input
  Saturation2 : Saturate  UpperLimit=UpperLimit  LowerLimit=LowerLimit  SampleTime=Ts
  Sum6 : Sum  InputSameDT=on  SaturateOnIntegerOverflow=on  SampleTime=Ts  OutDataTypeStr=Inherit: Same as first input
  Zero-Order Hold : ZeroOrderHold  SampleTime=Ts
  Out : Outport  SampleTime=Ts  InitialOutput=0  VectorParamsAs1DForOutWhenUnconnected=off
  wires:
  Zero-Order Hold/1 -> Sum6/1
  Saturation2/1 -> Out/1
  Discrete-Time Integrator/1 -> Sum6/2
  Kp4/1 -> Zero-Order Hold/1
  Kp5/1 -> Discrete-Time Integrator/1
  Sum6/1 -> Saturation2/1
  Error/1 -> Kp5/1, Kp4/1

== system Hybrid2_article_SVC_stage1/SVC Controller1/Firing Unit/Firing Unit CA/PLL sync on positive peak /Discrete PI Controller ==
  note: Discrete PID Controller
  note: Pierre Giroux, Gilbert Sybille
      | Power System Simulation Laboratory
      | IREQ, Hydro-Quebc
  Error : Inport  SampleTime=Ts
  Discrete-Time Integrator : DiscreteIntegrator  InitialCondition=Init  SampleTime=Ts  LimitOutput=on  UpperSaturationLimit=UpperLimit  LowerSaturationLimit=LowerLimit  ICPrevOutput=DiscIntNeverNeededParam  ICPrevScaledInput=DiscIntNeverNeededParam
  Kp4 : Gain  Gain=Kp  SaturateOnIntegerOverflow=on  SampleTime=Ts  OutDataTypeStr=Inherit: Same as input  ParamDataTypeStr=Inherit: Same as input
  Kp5 : Gain  Gain=Ki  SaturateOnIntegerOverflow=on  SampleTime=Ts  OutDataTypeStr=Inherit: Same as input  ParamDataTypeStr=Inherit: Same as input
  Saturation2 : Saturate  UpperLimit=UpperLimit  LowerLimit=LowerLimit  SampleTime=Ts
  Sum6 : Sum  InputSameDT=on  SaturateOnIntegerOverflow=on  SampleTime=Ts  OutDataTypeStr=Inherit: Same as first input
  Zero-Order Hold : ZeroOrderHold  SampleTime=Ts
  Out : Outport  SampleTime=Ts  InitialOutput=0  VectorParamsAs1DForOutWhenUnconnected=off
  wires:
  Zero-Order Hold/1 -> Sum6/1
  Saturation2/1 -> Out/1
  Discrete-Time Integrator/1 -> Sum6/2
  Kp4/1 -> Zero-Order Hold/1
  Kp5/1 -> Discrete-Time Integrator/1
  Sum6/1 -> Saturation2/1
  Error/1 -> Kp5/1, Kp4/1

== system Hybrid2_article_SVC_stage1/DFIG Wind Turbine/Control/Measurement and Transformation/Discrete 3-phase PLL-Driven Positive-Sequence Active & Reactive Power/Discrete 3-phase PLL-Driven Positive-Sequence Fundamental Value/Discrete Variable Frequency Mean value1 ==
  note: Pierre Giroux, Gilbert Sybille, Richard Gagnon
      | Power System Simulation Laboratory
      | IREQ, Hydro-Quebc
  note: Variable frequency - Discrete Mean Value
  Freq : Inport  PortDimensions=1
  In : Inport  Port=2  PortDimensions=1
  Correction subsystem : Subsystem
  Discrete Variable Transport Delay : Subsystem  mask(Discrete variable transport delay){MaxDelay=MaxDelay, InitialValue=0, Ts=Ts}
      mask prompts: MaxDelay "Maximum delay (s):"; InitialValue "Initial input:"; Ts "Sample time:"
      mask help:
      | Apply a delay to the first input (In) signal.
      | The second input (D) specifies the delay time.
  Gain : Gain  Gain=Ts  SaturateOnIntegerOverflow=on  OutDataTypeStr=Inherit: Same as input  ParamDataTypeStr=Inherit: Same as input
  Integ4 : DiscreteIntegrator  IntegratorMethod=Integration: Trapezoidal  SampleTime=Ts  ICPrevOutput=DiscIntNeverNeededParam  ICPrevScaledInput=DiscIntNeverNeededParam
  Number of samples per cycle : Fcn  Expr=1/u[1]/Ts
  Product : Product  InputSameDT=on  SaturateOnIntegerOverflow=on  OutDataTypeStr=Inherit: Same as first input
  Rounding Function : Rounding  Operator=ceil
  Step : Step  Time=1/Finit  SampleTime=Ts
  Sum5 : Sum  InputSameDT=on  SaturateOnIntegerOverflow=on  OutDataTypeStr=Inherit: Same as first input
  Sum7 : Sum  Inputs=-+  InputSameDT=on  SaturateOnIntegerOverflow=on  OutDataTypeStr=Inherit: Same as first input
  Switch : Switch  Threshold=0.5  SaturateOnIntegerOverflow=off
  To avoid division by zero : Saturate  UpperLimit=1e6  LowerLimit=1e-6
  Unit Delay : UnitDelay  InitialCondition=Vinit  SampleTime=Ts  HasFrameUpgradeWarning=on
  Mean : Outport  VectorParamsAs1DForOutWhenUnconnected=off
  wires:
  In/1 -> Integ4/1, Correction subsystem/3(In)  "In"
  Product/1 -> Sum5/1  "Mean value"
  Discrete Variable Transport Delay/1(Out) -> Sum7/1
  Sum7/1 -> Product/1
  Integ4/1 -> Discrete Variable Transport Delay/1(In), Sum7/2
  Freq/1 -> Product/2, To avoid division by zero/1  "Freq"
  Gain/1 -> Discrete Variable Transport Delay/2(D)  "Delay"
  Rounding Function/1 -> Gain/1, Correction subsystem/2(F)
  Number of samples per cycle/1 -> Rounding Function/1, Correction subsystem/1(N)
  Sum5/1 -> Switch/1
  Unit Delay/1 -> Switch/3
  Switch/1 -> Mean/1, Unit Delay/1
  To avoid division by zero/1 -> Number of samples per cycle/1  "Freq"
  Correction subsystem/1(Out) -> Sum5/2
  Step/1 -> Switch/2

== system Hybrid2_article_SVC_stage1/DFIG Wind Turbine/Control/Measurement and Transformation/Discrete 3-phase PLL-Driven Positive-Sequence Active & Reactive Power/Discrete 3-phase PLL-Driven Positive-Sequence Fundamental Value/Discrete Variable Frequency Mean value2 ==
  note: Variable frequency - Discrete Mean Value
  note: Pierre Giroux, Gilbert Sybille, Richard Gagnon
      | Power System Simulation Laboratory
      | IREQ, Hydro-Quebc
  Freq : Inport  PortDimensions=1
  In : Inport  Port=2  PortDimensions=1
  Correction subsystem : Subsystem
  Discrete Variable Transport Delay : Subsystem  mask(Discrete variable transport delay){MaxDelay=MaxDelay, InitialValue=0, Ts=Ts}
      mask prompts: MaxDelay "Maximum delay (s):"; InitialValue "Initial input:"; Ts "Sample time:"
      mask help:
      | Apply a delay to the first input (In) signal.
      | The second input (D) specifies the delay time.
  Gain : Gain  Gain=Ts  SaturateOnIntegerOverflow=on  OutDataTypeStr=Inherit: Same as input  ParamDataTypeStr=Inherit: Same as input
  Integ4 : DiscreteIntegrator  IntegratorMethod=Integration: Trapezoidal  SampleTime=Ts  ICPrevOutput=DiscIntNeverNeededParam  ICPrevScaledInput=DiscIntNeverNeededParam
  Number of samples per cycle : Fcn  Expr=1/u[1]/Ts
  Product : Product  InputSameDT=on  SaturateOnIntegerOverflow=on  OutDataTypeStr=Inherit: Same as first input
  Rounding Function : Rounding  Operator=ceil
  Step : Step  Time=1/Finit  SampleTime=Ts
  Sum5 : Sum  InputSameDT=on  SaturateOnIntegerOverflow=on  OutDataTypeStr=Inherit: Same as first input
  Sum7 : Sum  Inputs=-+  InputSameDT=on  SaturateOnIntegerOverflow=on  OutDataTypeStr=Inherit: Same as first input
  Switch : Switch  Threshold=0.5  SaturateOnIntegerOverflow=off
  To avoid division by zero : Saturate  UpperLimit=1e6  LowerLimit=1e-6
  Unit Delay : UnitDelay  InitialCondition=Vinit  SampleTime=Ts  HasFrameUpgradeWarning=on
  Mean : Outport  VectorParamsAs1DForOutWhenUnconnected=off
  wires:
  Step/1 -> Switch/2
  Correction subsystem/1(Out) -> Sum5/2
  To avoid division by zero/1 -> Number of samples per cycle/1  "Freq"
  Switch/1 -> Unit Delay/1, Mean/1
  Unit Delay/1 -> Switch/3
  Sum5/1 -> Switch/1
  Number of samples per cycle/1 -> Correction subsystem/1(N), Rounding Function/1
  Rounding Function/1 -> Correction subsystem/2(F), Gain/1
  Gain/1 -> Discrete Variable Transport Delay/2(D)  "Delay"
  Freq/1 -> To avoid division by zero/1, Product/2  "Freq"
  Integ4/1 -> Sum7/2, Discrete Variable Transport Delay/1(In)
  Sum7/1 -> Product/1
  Discrete Variable Transport Delay/1(Out) -> Sum7/1
  Product/1 -> Sum5/1  "Mean value"
  In/1 -> Correction subsystem/3(In), Integ4/1  "In"
